simulink model "dpt_detaliz"  (R2021b)
settings: Solver=VariableStepAuto  StartTime=0.0  StopTime=0.5  RelTol=1e-3
values from neighbouring files (symbols this model uses):
  Jn = 2*Jd    (= 3.92e-05)    [pasport_dpt.m]
  ke = (Un-R*In)/wn    (= 0.236312997347)    [pasport_dpt.m]
  km = Mn/In    (= 0.156097560976)    [pasport_dpt.m]
  ku = 20    [pasport_dpt.m]
  L = 10^-3*140    (= 0.14)    [pasport_dpt.m]
  R = 51    [pasport_dpt.m]
settings Model: Creator=Admin  LastModifiedBy=Admin
settings SolverCC: AlgebraicLoopSolver=TrustRegion
settings DebuggingCC: SFMachineParentedDataDiag=warning

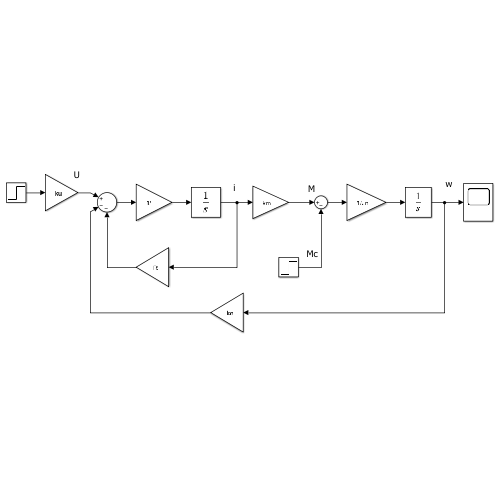
[thumbnail: Simulink's stored preview of the top-level diagram]
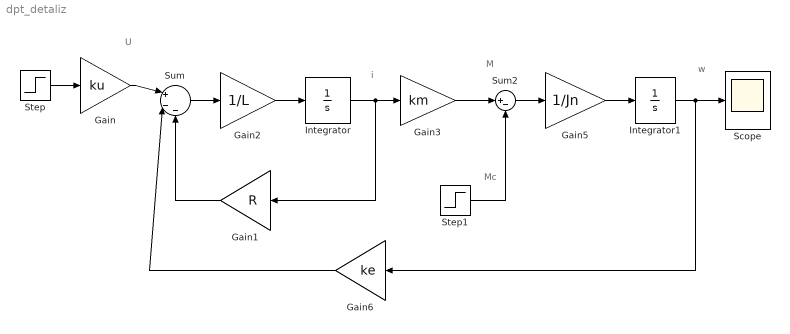
== system dpt_detaliz ==
  note: Mc
  note: M
  note: w
  note: i
  note: U
  Gain : Gain  Gain=ku
  Gain1 : Gain  Gain=R
  Gain2 : Gain  Gain=1/L
  Gain3 : Gain  Gain=km
  Gain5 : Gain  Gain=1/Jn
  Gain6 : Gain  Gain=ke
  Integrator : Integrator
  Integrator1 : Integrator
  Scope : Scope
  Step : Step  Time=0  SampleTime=0
  Step1 : Step  Time=0.35  After=0.02  SampleTime=0
  Sum : Sum  Inputs=|+--
  Sum2 : Sum  Inputs=|+-
  wires:
  Step/1 -> Gain/1
  Gain/1 -> Sum/1
  Sum/1 -> Gain2/1
  Gain2/1 -> Integrator/1
  Gain1/1 -> Sum/3
  Integrator/1 -> Gain1/1, Gain3/1
  Gain3/1 -> Sum2/1
  Integrator1/1 -> Gain6/1, Scope/1
  Gain5/1 -> Integrator1/1
  Gain6/1 -> Sum/2
  Sum2/1 -> Gain5/1
  Step1/1 -> Sum2/2
